simulink model "Plant"  (R2025b)
settings: Solver=VariableStepAuto  StartTime=0.0  StopTime=10.0  RelTol=1e-3
values from neighbouring files (symbols this model uses):
  alpha_deg = data(:, 1)    [init.m]
  cl_data = data(:, 2)    [init.m]
  D_heave = 500    [init.m]
  m = 585    [init.m]
  q_S = 0.5 * rho * V_takeoff^2 * S_total    (= 42708.5041668)    [init.m]
  sensor_sample_time = 1 / height_sensor_freq    (= 0.1)    [init.m]
  servo_max_speed = deg2rad(servo_speed_deg_sec)    [init.m]
  start_height = 0.1    [init.m]
settings Model: Creator=parks  LastModifiedBy=parks

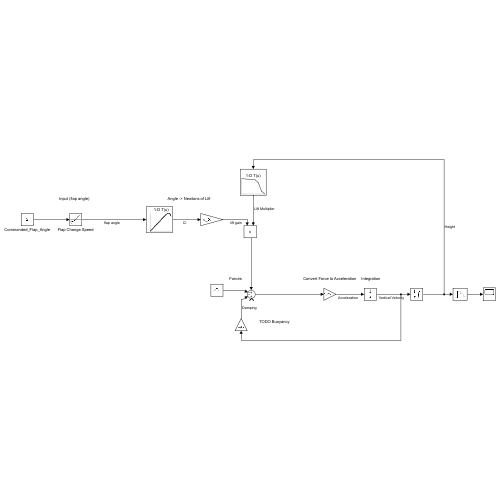
[thumbnail: Simulink's stored preview of the top-level diagram]
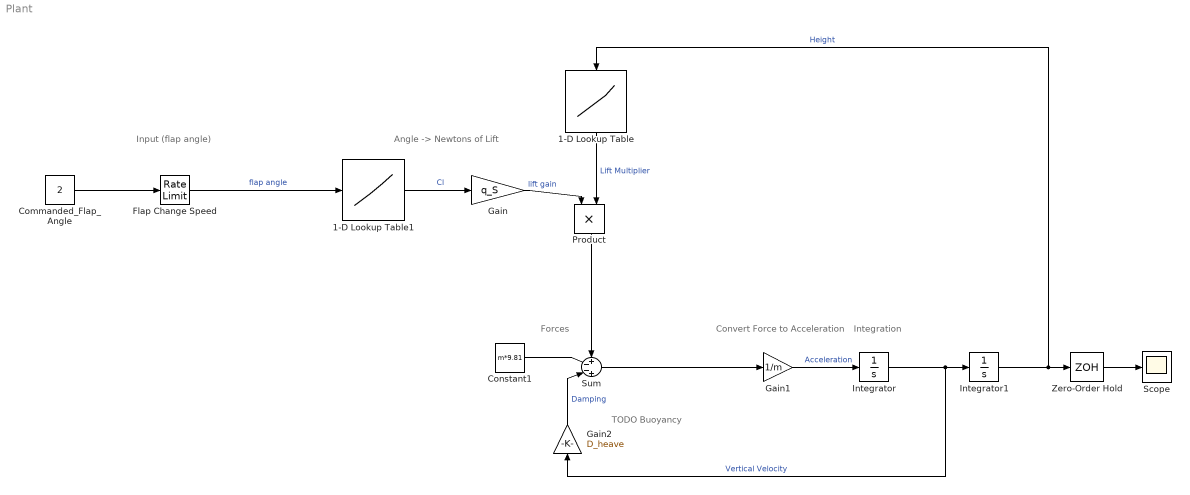
== system Plant ==
  note: TODO Buoyancy
  note: Integration
  note: Convert Force to Acceleration
  note: Forces
  note: Input (flap angle)
  note: Angle -> Newtons of Lift
  1-D Lookup Table : Lookup_n-D  NumberOfTableDimensions=1  BreakpointsForDimension1=[0, 0.4, 0.5, 0.6, 0.7]  Table=[1.1, 1.0, 0.8, 0.2, 0.0]  InternalRulePriority=Speed  RndMeth=Simplest
  1-D Lookup Table1 : Lookup_n-D  NumberOfTableDimensions=1  BreakpointsForDimension1=alpha_deg  Table=cl_data  InternalRulePriority=Speed  RndMeth=Simplest
  Commanded_Flap_Angle : Constant  Value=2
  Constant1 : Constant  Value=m*9.81
  Flap Change Speed : RateLimiter  RisingSlewLimit=servo_max_speed  FallingSlewLimit=-servo_max_speed  SampleTimeMode=inherited
  Gain : Gain  Gain=q_S
  Gain1 : Gain  Gain=1/m
  Gain2 : Gain  Gain=D_heave
  Integrator : Integrator
  Integrator1 : Integrator  InitialCondition=start_height  LimitOutput=on  LowerSaturationLimit=0
  Product : Product
  Scope : Scope
      settings: ActiveDisplayYMinimum=0.075647594713752209  ActiveDisplayYMaximum=0.76754445137472849
  Sum : Sum  Inputs=+--+
  Zero-Order Hold : ZeroOrderHold  SampleTime=sensor_sample_time
  wires:
  Commanded_Flap_Angle/1 -> Flap Change Speed/1
  Flap Change Speed/1 -> 1-D Lookup Table1/1  "flap angle"
  Gain/1 -> Product/1  "lift gain"
  Constant1/1 -> Sum/2
  Sum/1 -> Gain1/1
  Gain1/1 -> Integrator/1  "Acceleration"
  Integrator/1 -> Gain2/1, Integrator1/1  "Vertical Velocity"
  Integrator1/1 -> 1-D Lookup Table/1, Zero-Order Hold/1  "Height"
  Zero-Order Hold/1 -> Scope/1
  1-D Lookup Table/1 -> Product/2  "Lift Multiplier"
  Product/1 -> Sum/1
  Gain2/1 -> Sum/3  "Damping"
  1-D Lookup Table1/1 -> Gain/1  "Cl"
